simulink model "Comunicacion_serie_"  (R2017a)
settings: Solver=VariableStepAuto  StartTime=0.0  StopTime=inf  RelTol=1e-3
undefined symbols (not defined in the file or in its folder): serial
libraries: instrumentlib x3
settings Model: Creator=Federico  LastModifiedBy=Martin

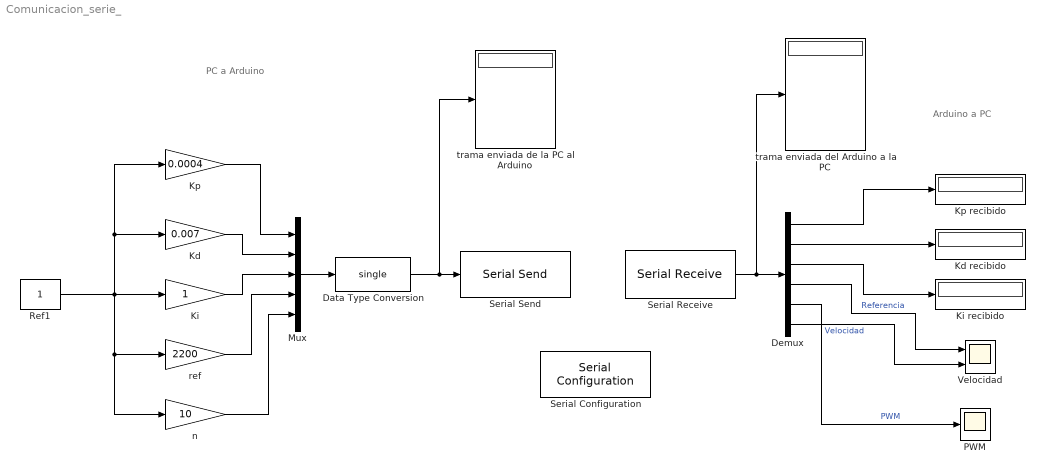
== system Comunicacion_serie_ ==
  note: Arduino a PC
  note: PC a Arduino
  Data Type Conversion : DataTypeConversion  OutDataTypeStr=single
  Demux : Demux  Outputs=6
  Kd : Gain  Gain=0.007
  Kd recibido : Display
  Ki : Gain
  Ki recibido : Display
  Kp : Gain  Gain=0.0004
  Kp recibido : Display
  Mux : Mux  Inputs=5
  PWM : Scope
  Ref1 : Constant  OutDataTypeStr=single  SampleTime=1
  Serial Configuration : instrumentlib/Serial Configuration  Priority=-200000  ComPortMenu=<Please select a port...>  ComPort=COM4  ObjConstructor=serial('COM4');  BaudRate=9600  DataBits=8  Parity=none  StopBits=1  FlowControl=none  Timeout=10  ByteOrder=LittleEndian
  Serial Receive : instrumentlib/Serial Receive  ComPortMenu=<Please select a port...>  ComPort=COM4  ObjConstructor=serial('COM4');  Header=efgh  Terminator=<none>  DataSize="[1  6]"  DataType=single  EnableBlockingMode=on  ActionDataUnavailable=Output last received value  CustomValue=0  SampleTime=1
  Serial Send : instrumentlib/Serial Send  ComPortMenu=<Please select a port...>  ComPort=COM4  ObjConstructor=serial('COM4');  Header=abcd  Terminator=<none>  EnableBlockingMode=on
  Velocidad : Scope  NumInputPorts=2
  n : Gain  Gain=10
  ref : Gain  Gain=2200
  "trama enviada de la PC al Arduino " : Display
  trama enviada del Arduino a la PC : Display
  wires:
  Serial Receive/1 -> trama enviada del Arduino a la PC/1, Demux/1
  Demux/1 -> Kp recibido/1
  Demux/2 -> Kd recibido/1
  Demux/3 -> Ki recibido/1
  Demux/4 -> Velocidad/1  "Referencia"
  Demux/6 -> Velocidad/2  "Velocidad"
  Demux/5 -> PWM/1  "PWM"
  Data Type Conversion/1 -> "trama enviada de la PC al Arduino "/1, Serial Send/1
  Mux/1 -> Data Type Conversion/1
  Kp/1 -> Mux/1
  Kd/1 -> Mux/2
  Ki/1 -> Mux/3
  ref/1 -> Mux/4
  n/1 -> Mux/5
  Ref1/1 -> n/1, ref/1, Kp/1, Kd/1, Ki/1
